simulink library "nmc"  (R2015b)
settings: Solver=ode45  SolverMode=SingleTasking  StartTime=0.0  StopTime=10.0  RelTol=1e-3
undefined symbols (not defined in the file): AnkleStance, AnkleSwing, c, c_jointstop, CtrlPar_FP_List, CtrlPar_FP_R_List, CtrlPar_LL_List, CtrlPar_St_List, CtrlPar_St_R_List, CtrlPar_Sw_List, CtrlPar_Sw_R_List, CtrlPar_theta0_List, CtrlPar_Tr_List, CtrlPar_Tr_R_List, CtrlPar_VelocityFile_List, D1G_HAT, eref, FmaxBFSH, FmaxGAS, FmaxGLU, FmaxHAB, FmaxHAD, FmaxHAM, FmaxHFL, FmaxRF, FmaxSOL, FmaxTA, FmaxVAS, init_a_tgt, init_a_tgtR, K, leg_l, LongDelay, LongLoopDelay, loptBFSH, loptGAS, loptGLU, loptHAB, loptHAD, loptHAM, loptHFL, loptRF, loptSOL, loptTA, loptVAS, lslackBFSH, lslackGAS, lslackGLU, lslackHAB, lslackHAD, lslackHAM, lslackHFL, lslackRF, lslackSOL, lslackTA, lslackVAS, magnitude, maxLoad_control_List, MeanStepsAnkle, MidDelay ... (+99)
libraries: nmc x63, simulink x31, simulink_extras x30, LopesDevelopmentLibrary x3
(part 10 of 10)

== system nmc/NMC Model/Neural Control Layer (Spinal Cord Control)/R Swing Phase (sagittal)/kneeii_damp and hold &kneeiii_leg stop &kneeiv_stance preparation/kneeii_damp and hold ==
  note: Knee Phase i
  CtrlPar : Inport
  a_tgt : Inport  Port=2
  VceVAS : Inport  Port=3
  VceBFSH : Inport  Port=4
  VceRF : Inport  Port=5
  LceRF : Inport  Port=6
  Enable : EnablePort  StatesWhenEnabling=reset  ZeroCross=off
  Constant5 : Constant
  Demux2 : Demux  Outputs=5
  Divide1 : Product
  Divide2 : Product  Inputs=3
  Divide3 : Product  Inputs=*/
  Divide4 : Product  Inputs=*/
  Divide5 : Product
  Divide6 : Product
  Divide7 : Product  Inputs=*/
  Sum1 : Sum  Inputs=|-+  SaturateOnIntegerOverflow=on  InputSameDT=on  OutDataTypeStr=Inherit: Same as first input
  Sum10 : Sum  Inputs=|++  SaturateOnIntegerOverflow=on  InputSameDT=on  OutDataTypeStr=Inherit: Same as first input
  Sum2 : Sum  Inputs=|-+  SaturateOnIntegerOverflow=on  InputSameDT=on  OutDataTypeStr=Inherit: Same as first input
  Sum7 : Sum  Inputs=|++  SaturateOnIntegerOverflow=on  InputSameDT=on  OutDataTypeStr=Inherit: Same as first input
  positive half{,1..3} (4 alike) : Saturate  UpperLimit=inf  LowerLimit=0  ZeroCross=off
  SRF_Sw_kii : Outport  OutputWhenDisabled=reset  InitialOutput=0
  SBFSH_Sw_kii : Outport  Port=2  OutputWhenDisabled=reset  InitialOutput=0
  wires:
  CtrlPar/1 -> Demux2/1
  Demux2/1 -> Divide5/2  "VGainVAS_RF"
  VceBFSH/1 -> positive half/1, Divide3/1
  Divide5/1 -> SRF_Sw_kii/1
  positive half3/1 -> Divide5/1
  positive half/1 -> Divide1/1
  Demux2/2 -> Divide1/2  "VGainBFSH"
  Divide1/1 -> Divide2/1
  positive half1/1 -> Divide2/2
  Demux2/3 -> Divide3/2  "phi2lopt_BFSH"
  VceRF/1 -> Divide4/1
  Demux2/4 -> Divide4/2, Divide6/1, Divide7/2  "a2lopt_RF"
  Sum7/1 -> positive half1/1
  positive half2/1 -> Divide2/3
  a_tgt/1 -> Sum1/2
  Demux2/5 -> Sum1/1  "aRef_RF"
  Sum1/1 -> Divide6/2
  Divide6/1 -> Sum10/1
  Constant5/1 -> Sum10/2
  Sum10/1 -> Sum2/1  "lceOffRF"
  LceRF/1 -> Sum2/2
  Sum2/1 -> Divide7/1
  Divide7/1 -> positive half2/1
  Divide2/1 -> SBFSH_Sw_kii/1
  VceVAS/1 -> positive half3/1
  Divide3/1 -> Sum7/1
  Divide4/1 -> Sum7/2

== system nmc/NMC Model/Neural Control Layer (Spinal Cord Control)/R Swing Phase (sagittal)/kneeii_damp and hold &kneeiii_leg stop &kneeiv_stance preparation/kneeiii_leg stop ==
  note: Knee Phase iii
  CtrlPar : Inport
  a_tgt : Inport  Port=2
  LceHAM : Inport  Port=3
  Enable : EnablePort  StatesWhenEnabling=reset  ZeroCross=off
  Constant5 : Constant
  Demux1 : Demux  Outputs=7
  Divide{1..2,5,22} (4 alike) : Product
  Sum1 : Sum  Inputs=-+|  SaturateOnIntegerOverflow=on  InputSameDT=on  OutDataTypeStr=Inherit: Same as first input
  Sum10 : Sum  Inputs=+-|  SaturateOnIntegerOverflow=on  InputSameDT=on  OutDataTypeStr=Inherit: Same as first input
  Sum2 : Sum  Inputs=++|  SaturateOnIntegerOverflow=on  InputSameDT=on  OutDataTypeStr=Inherit: Same as first input
  Sum3 : Sum  Inputs=+-|  SaturateOnIntegerOverflow=on  InputSameDT=on  OutDataTypeStr=Inherit: Same as first input
  Sum4 : Sum  Inputs=+-|  SaturateOnIntegerOverflow=on  InputSameDT=on  OutDataTypeStr=Inherit: Same as first input
  positive half1 : Saturate  UpperLimit=inf  LowerLimit=0  ZeroCross=off
  positive half2 : Saturate  UpperLimit=inf  LowerLimit=0  ZeroCross=off
  SHAM_Sw_kiii : Outport  OutputWhenDisabled=reset  InitialOutput=0
  SKFL_Sw_kiii : Outport  Port=2  OutputWhenDisabled=reset  InitialOutput=0
  SGAS_Sw_kiii : Outport  Port=3  OutputWhenDisabled=reset  InitialOutput=0
  wires:
  CtrlPar/1 -> Demux1/1
  Sum1/1 -> positive half2/1  "del_LceMAN"
  LceHAM/1 -> Sum1/2  "LceHAM"
  positive half2/1 -> Divide5/1  "del_lce"
  Constant5/1 -> Sum10/1
  Divide22/1 -> Sum10/2
  a_tgt/1 -> Sum2/1
  Demux1/1 -> Sum2/2  "a_del"
  Sum2/1 -> Sum3/1  "a_thr"
  Demux1/2 -> Sum3/2  "aRef_HAM"
  Sum3/1 -> Divide22/1
  Demux1/3 -> Divide22/2  "a2lopt_HAM"
  Sum10/1 -> Sum1/1  "lceOffHAM"
  Demux1/4 -> Divide5/2  "LGainHAM"
  Divide5/1 -> Sum4/1, SHAM_Sw_kiii/1  "S_HAM"
  Sum4/1 -> positive half1/1
  Demux1/5 -> Sum4/2  "SHAM_thr"
  positive half1/1 -> Divide1/1, Divide2/1
  Demux1/6 -> Divide1/2  "SGainHAM_KFL"
  Divide1/1 -> SKFL_Sw_kiii/1
  Divide2/1 -> SGAS_Sw_kiii/1
  Demux1/7 -> Divide2/2  "SGainHAM_GAS"

== system nmc/NMC Model/Neural Control Layer (Spinal Cord Control)/R Swing Phase (sagittal)/kneeii_damp and hold &kneeiii_leg stop &kneeiv_stance preparation/kneeiv_stance preparation ==
  note: Knee Phase iii
  CtrlPar : Inport
  a_tgt : Inport  Port=2
  LceHFL : Inport  Port=3
  lceGLU : Inport  Port=4
  lceVAS : Inport  Port=5
  Enable : EnablePort  StatesWhenEnabling=reset  ZeroCross=off
  Constant1 : Constant
  Constant2 : Constant
  Constant5 : Constant  Value=pi/2
  Demux2 : Demux  Outputs=8
  Divide{1..3,5..6} (5 alike) : Product
  Sum1 : Sum  Inputs=-+|  SaturateOnIntegerOverflow=on  InputSameDT=on  OutDataTypeStr=Inherit: Same as first input
  Sum2 : Sum  Inputs=++|  SaturateOnIntegerOverflow=on  InputSameDT=on  OutDataTypeStr=Inherit: Same as first input
  Sum3 : Sum  Inputs=+-|  SaturateOnIntegerOverflow=on  InputSameDT=on  OutDataTypeStr=Inherit: Same as first input
  Sum4 : Sum  Inputs=+-|  SaturateOnIntegerOverflow=on  InputSameDT=on  OutDataTypeStr=Inherit: Same as first input
  Sum5 : Sum  Inputs=++|  SaturateOnIntegerOverflow=on  InputSameDT=on  OutDataTypeStr=Inherit: Same as first input
  Sum6 : Sum  Inputs=-+|  SaturateOnIntegerOverflow=on  InputSameDT=on  OutDataTypeStr=Inherit: Same as first input
  Sum7 : Sum  Inputs=+-|  SaturateOnIntegerOverflow=on  InputSameDT=on  OutDataTypeStr=Inherit: Same as first input
  Sum9 : Sum  Inputs=-+|  SaturateOnIntegerOverflow=on  InputSameDT=on  OutDataTypeStr=Inherit: Same as first input
  positive half1 : Saturate  UpperLimit=inf  LowerLimit=0  ZeroCross=off
  positive half2 : Saturate  UpperLimit=inf  LowerLimit=0  ZeroCross=off
  positive half3 : Saturate  UpperLimit=inf  LowerLimit=0  ZeroCross=off
  SHFL_Sw_kiv : Outport  OutputWhenDisabled=reset  InitialOutput=0
  SGLU_Sw_kiv : Outport  Port=2  OutputWhenDisabled=reset  InitialOutput=0
  SVAS_Sw_kiv : Outport  Port=3  OutputWhenDisabled=reset  InitialOutput=0
  wires:
  CtrlPar/1 -> Demux2/1
  Sum1/1 -> positive half2/1
  LceHFL/1 -> Sum1/2
  positive half2/1 -> Divide5/1
  a_tgt/1 -> Sum2/2
  Constant5/1 -> Sum2/1
  Demux2/1 -> Sum3/2  "phiRef_HFL"
  Sum2/1 -> Sum3/1, Sum4/1
  Sum3/1 -> Divide1/1
  Demux2/2 -> Divide1/2  "phi2lopt_HFL"
  Demux2/5 -> Divide2/2  "phi2lopt_GLU"
  Demux2/4 -> Sum4/2  "phiRef_GLU"
  Sum4/1 -> Divide2/1
  Demux2/3 -> Divide5/2  "LGainHFL"
  Divide5/1 -> SHFL_Sw_kiv/1
  Constant1/1 -> Sum5/1
  Divide1/1 -> Sum5/2
  Sum5/1 -> Sum1/1  "lceOffHFL"
  Sum6/1 -> positive half1/1  "del_lce"
  lceGLU/1 -> Sum6/2  "lceGLU"
  positive half1/1 -> Divide3/1
  Demux2/6 -> Divide3/2  "LGainGLU"
  Divide3/1 -> SGLU_Sw_kiv/1
  Constant2/1 -> Sum7/1
  Divide2/1 -> Sum7/2
  Sum7/1 -> Sum6/1  "lceOffGLU"
  Sum9/1 -> positive half3/1
  lceVAS/1 -> Sum9/2
  positive half3/1 -> Divide6/1
  Divide6/1 -> SVAS_Sw_kiv/1
  Demux2/7 -> Sum9/1  "loffVAS"
  Demux2/8 -> Divide6/2  "LGainVAS"

== stateflow chart nmc/LopesToGeyer_angles/AnklePredictorLeft/LeftStance/Frequency  ==
  state PurePos
    entry:
    count = count +1;
    mean_freq = mean_freq*(N-1)/N + (1/N) * freq;
  state SWITCH
    entry:
    start_time = time_sig;
    exit:
    freq =1/(time_sig-start_time);
  state Start
    entry:
    mean_freq = 0;
    count = 0;
  SWITCH -> PurePos : [InSig==0]
  PurePos -> SWITCH : [InSig==1]
  (default) -> Start
  Start -> SWITCH : [InSig == 1]
  data: time_sig input; start_time local; InSig input; count output; mean_freq output; N input; freq local

== matlab function nmc/ParamScaling/ScalerFull ==
  data: ParamFile input; ScaledParam output; VelocityFile input; Velocity input
function ScaledParam  = GetParams(ParamFile,VelocityFile,Velocity)

%#codegen
% This Function is able to scale the NMC parameters based on the current
% velocity. Scaling is done linearly.

%% Turning Matrix in case of one row (data is treated as a row vector instead of a column vector in that case)
if length(VelocityFile) == 1
    ScaledParam = ParamFile;
else 
    %% PreAllocation
    ScaledParam = zeros(1,size(ParamFile(1,:),2));
    
    %% Sorting the velocity and the  parameter files
    [VelocityFile,sortIndex] = sort(VelocityFile);
    ParamFile = ParamFile(sortIndex,:);
    
    %% Finding the two currently active parameter sets
    a1 = find(Velocity>VelocityFile,1,'last');
    a2 = find(Velocity<VelocityFile,1,'first');
    
    if isempty(a1)
        % If a1 is empty, the velocity is lower than the lowest velocity
        % known. In that case, the parameters belonging to the lowest
        % parameterset are chosen
        ScaledParam(1,:) = ParamFile(1,:);
    elseif isempty(a2)
        % If a2 is empty, the velocity is higher than the highest velocity
        % known. In that case, the parameters belonging to the highest
        % parameterset are chosen
        ScaledParam(1,:) = ParamFile(end,:);
    else
        % Linear scaling between two paramSets
        linGain = (Velocity - VelocityFile(a1))/(VelocityFile(a2) - VelocityFile(a1));
        ScaledParam(1,:) = ParamFile(a2(1),:).*linGain(1) + ParamFile(a1(1),:).*(1-linGain(1));
    end
end
end

== matlab function nmc/LopesToGeyer_angles/AnklePredictorLeft/Shape estimator left/Phase 2/Oscillator shape Bias/ROC_Estimate ==
  data: shape input; output output; freq input; t input
function output  = roc_est(shape,freq,t)
%% Pre-allocating
N = size(shape,2);
M = size(shape,1);
output = zeros(M,1);

%% Estimating current indices in Shape

%% Estimating current index in shape
ind = 1 + (N-1)*t*freq;

%% Flooring and finding diff
ind_fl = floor(ind);
int_diff = ind-ind_fl;

%% Setting bounds
if ind > N
    ind = N;
    ind_fl = N;
end
assert(ind_fl<N+1) 
assert(ind_fl>0);

%% Calculating shape
ind_l = zeros(1,2);
ind_l(1,:) = ind_fl:ind_fl+1;
if ind_l(end) <= N
    angle = zeros(M,1);
    angle(:,1) = interp1(ind_l,shape(:,ind_l)',ind_l(1)+int_diff)';
else
    angle = shape(:,N);
end 

%% Output
output(:,1) = angle;
end

== matlab function nmc/LopesToGeyer_angles/AnklePredictorLeft/Shape estimator left/Phase 1/Oscillator shape Bias/ROC_Estimate ==
  data: shape input; output output; freq input; t input
function output  = roc_est(shape,freq,t)
%% Pre-allocating
N = size(shape,2);
M = size(shape,1);
output = zeros(M,1);

%% Estimating current indices in Shape

%% Estimating current index in shape
ind = 1 + (N-1)*t*freq;

%% Flooring and finding diff
ind_fl = floor(ind);
int_diff = ind-ind_fl;

%% Setting bounds
if ind > N
    ind = N;
    ind_fl = N;
end
assert(ind_fl<N+1) 
assert(ind_fl>0);

%% Calculating shape
ind_l = zeros(1,2);
ind_l(1,:) = ind_fl:ind_fl+1;
if ind_l(end) <= N
    angle = zeros(M,1);
    angle(:,1) = interp1(ind_l,shape(:,ind_l)',ind_l(1)+int_diff)';
else
    angle = shape(:,N);
end 

%% Output
output(:,1) = angle;
end

== stateflow chart nmc/LopesToGeyer_angles/AnklePredictorLeft/LeftStance1/Frequency  ==
  state PurePos
    entry:
    count = count +1;
    mean_freq = mean_freq*(N-1)/N + (1/N) * freq;
  state SWITCH
    entry:
    start_time = time_sig;
    exit:
    freq =1/(time_sig-start_time);
  state Start
    entry:
    mean_freq = 0;
    count = 0;
  SWITCH -> PurePos : [InSig==0]
  PurePos -> SWITCH : [InSig==1]
  (default) -> Start
  Start -> SWITCH : [InSig == 1]
  data: time_sig input; start_time local; InSig input; count output; mean_freq output; N input; freq local

== stateflow chart nmc/LopesToGeyer_angles/AnklePredictorRight/LeftSwing/Frequency  ==
  state PurePos
    entry:
    count = count +1;
    mean_freq = mean_freq*(N-1)/N + (1/N) * freq;
  state SWITCH
    entry:
    start_time = time_sig;
    exit:
    freq =1/(time_sig-start_time);
  state Start
    entry:
    mean_freq = 0;
    count = 0;
  SWITCH -> PurePos : [InSig==0]
  PurePos -> SWITCH : [InSig==1]
  (default) -> Start
  Start -> SWITCH : [InSig == 1]
  data: time_sig input; start_time local; InSig input; count output; mean_freq output; N input; freq local

== stateflow chart nmc/LopesToGeyer_angles/AnklePredictorRight/LeftStance/Frequency  ==
  state PurePos
    entry:
    count = count +1;
    mean_freq = mean_freq*(N-1)/N + (1/N) * freq;
  state SWITCH
    entry:
    start_time = time_sig;
    exit:
    freq =1/(time_sig-start_time);
  state Start
    entry:
    mean_freq = 0;
    count = 0;
  SWITCH -> PurePos : [InSig==0]
  PurePos -> SWITCH : [InSig==1]
  (default) -> Start
  Start -> SWITCH : [InSig == 1]
  data: time_sig input; start_time local; InSig input; count output; mean_freq output; N input; freq local

== matlab function nmc/LopesToGeyer_angles/AnklePredictorRight/Shape estimator left/Phase 1/Oscillator shape Bias/ROC_Estimate ==
  data: shape input; output output; freq input; t input
function output  = roc_est(shape,freq,t)
%% Pre-allocating
N = size(shape,2);
M = size(shape,1);
output = zeros(M,1);

%% Estimating current indices in Shape

%% Estimating current index in shape
ind = 1 + (N-1)*t*freq;

%% Flooring and finding diff
ind_fl = floor(ind);
int_diff = ind-ind_fl;

%% Setting bounds
if ind > N
    ind = N;
    ind_fl = N;
end
assert(ind_fl<N+1) 
assert(ind_fl>0);

%% Calculating shape
ind_l = zeros(1,2);
ind_l(1,:) = ind_fl:ind_fl+1;
if ind_l(end) <= N
    angle = zeros(M,1);
    angle(:,1) = interp1(ind_l,shape(:,ind_l)',ind_l(1)+int_diff)';
else
    angle = shape(:,N);
end 

%% Output
output(:,1) = angle;
end

== matlab function nmc/LopesToGeyer_angles/AnklePredictorRight/Shape estimator left/Phase 2/Oscillator shape Bias/ROC_Estimate ==
  data: shape input; output output; freq input; t input
function output  = roc_est(shape,freq,t)
%% Pre-allocating
N = size(shape,2);
M = size(shape,1);
output = zeros(M,1);

%% Estimating current indices in Shape

%% Estimating current index in shape
ind = 1 + (N-1)*t*freq;

%% Flooring and finding diff
ind_fl = floor(ind);
int_diff = ind-ind_fl;

%% Setting bounds
if ind > N
    ind = N;
    ind_fl = N;
end
assert(ind_fl<N+1) 
assert(ind_fl>0);

%% Calculating shape
ind_l = zeros(1,2);
ind_l(1,:) = ind_fl:ind_fl+1;
if ind_l(end) <= N
    angle = zeros(M,1);
    angle(:,1) = interp1(ind_l,shape(:,ind_l)',ind_l(1)+int_diff)';
else
    angle = shape(:,N);
end 

%% Output
output(:,1) = angle;
end
